simulink model "q1"  (R2019b)
settings: Solver=VariableStepAuto  StartTime=0.0  StopTime=10.0  RelTol=1e-3
settings Model: Creator=nrjbs  LastModifiedBy=nrjbs

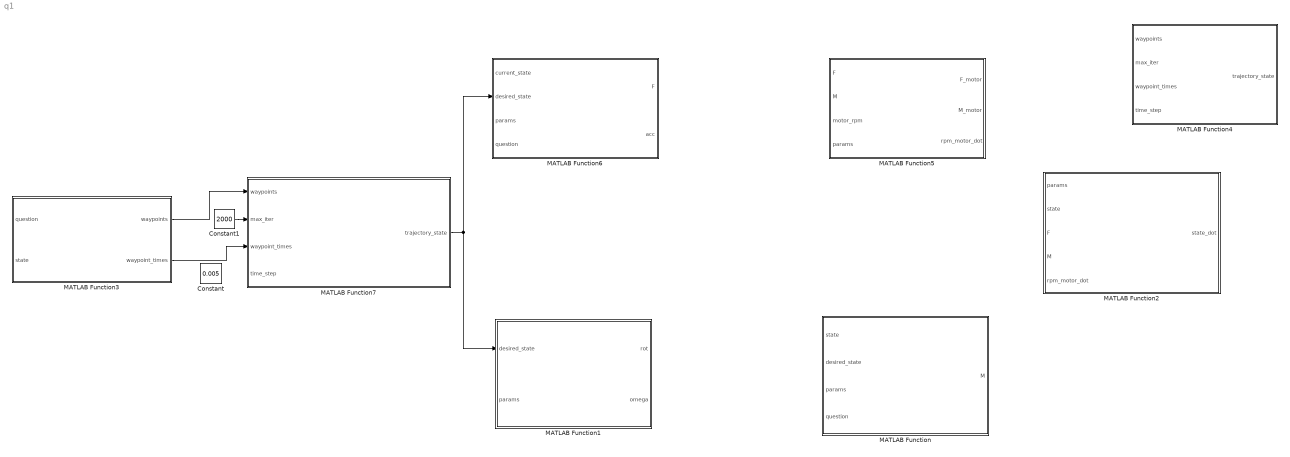
== system q1 ==
  Constant : Constant  Value=0.005
  Constant1 : Constant  Value=2000
  MATLAB Function : MATLAB Function  TreatAsAtomicUnit=on
  MATLAB Function1 : MATLAB Function  TreatAsAtomicUnit=on
  MATLAB Function2 : MATLAB Function  TreatAsAtomicUnit=on
  MATLAB Function3 : MATLAB Function  TreatAsAtomicUnit=on
  MATLAB Function4 : MATLAB Function  TreatAsAtomicUnit=on
  MATLAB Function5 : MATLAB Function  TreatAsAtomicUnit=on
  MATLAB Function6 : MATLAB Function  TreatAsAtomicUnit=on
  MATLAB Function7 : MATLAB Function  TreatAsAtomicUnit=on
  wires:
  MATLAB Function3/1(waypoints) -> MATLAB Function7/1(waypoints)
  MATLAB Function3/2(waypoint_times) -> MATLAB Function7/3(waypoint_times)
  Constant1/1 -> MATLAB Function7/2(max_iter)
  MATLAB Function7/1(trajectory_state) -> MATLAB Function6/2(desired_state), MATLAB Function1/1(desired_state)

== matlab function q1/MATLAB Function1 ==
  data: desired_state input; rot output; params input; omega output
function [rot, omega] = attitude_planner(desired_state, params)

== matlab function q1/MATLAB Function ==
  data: state input; M output; desired_state input; params input; question input
function M  = attitude_controller(state,desired_state,params,question)

== matlab function q1/MATLAB Function2 ==
  data: params input; state_dot output; state input; F input; M input; rpm_motor_dot input
function state_dot  = dynamics(params, state, F, M, rpm_motor_dot)
% Input parameters

== matlab function q1/MATLAB Function3 ==
  data: question input; waypoints output; state input; waypoint_times output
function [waypoints, waypoint_times] = lookup_waypoints(question, state)

== matlab function q1/MATLAB Function4 ==
  data: waypoints input; trajectory_state output; max_iter input; waypoint_times input; time_step input
function trajectory_state = trajectory_planner(waypoints, max_iter, waypoint_times, time_step)

== matlab function q1/MATLAB Function5 ==
  data: F input; F_motor output; M input; motor_rpm input; params input; M_motor output; rpm_motor_dot output
function [F_motor,M_motor,rpm_motor_dot] = motor_model(F,M,motor_rpm,params)

== matlab function q1/MATLAB Function6 ==
  data: current_state input; F output; desired_state input; params input; question input; acc output
function [F, acc] = position_controller(current_state, desired_state, params, question)

== matlab function q1/MATLAB Function7 ==
  data: waypoints input; trajectory_state output; max_iter input; waypoint_times input; time_step input
function trajectory_state = trajectory_planner(waypoints, max_iter, waypoint_times, time_step)
